simulink model "FinalmodelMad2Order"  (R2022b)
settings: Solver=FixedStepAuto  StartTime=0.0  StopTime=inf  RelTol=1e-3  EnableMultiTasking=on
libraries: vexarmcortexlib x25, vexcommonlib x1
settings Model: ExtModeTrigDuration=25  Creator=Mihai Nicoara  LastModifiedBy=bobsi
settings SolverCC: AutoInsertRateTranBlk=on
settings OptimizationCC: EnhancedBackFolding=on  PassReuseOutputArgsAs=Individual arguments  ZeroExternalMemoryAtStartup=off  ZeroInternalMemoryAtStartup=off  MaxStackSize=64  OptimizeBlockOrder=speed  DifferentSizesBufferReuse=on  OptimizationCustomize=off  EfficientTunableParamExpr=on
settings DebuggingCC: ParameterTunabilityLossMsg=error
settings HardwareCC: ProdBitPerPointer=32  ProdBitPerSizeT=32  ProdBitPerPtrDiffT=32  ProdLargestAtomicInteger=Long  ProdLargestAtomicFloat=Double  ProdWordSize=32  ProdHWDeviceType=ARM Compatible->ARM Cortex
settings SFSimCC: MATLABDynamicMemAlloc=off
settings RTWCC: Description=Embedded Coder  SystemTargetFile=ert.tlc  HardwareBoard=ARM Cortex-based VEX Microcontroller  TLCOptions="-aInlineSetEventsForThisBaseRateFcn=TLC_FALSE -aSuppressMultiTaskScheduler=TLC_FALSE  -aRateBasedStepFcn=0"  TemplateMakefile=ert_default_tmf  Toolchain=GNU Tools for VEX ARM Cortex
settings CodeAppCC: ForceParamTrailComments=on  IgnoreCustomStorageClasses=off  OperatorAnnotations=on  SimulinkDataObjDesc=on  SFDataObjDesc=on  InsertBlockDesc=on
settings ERTTargetCC: ExtModeTransport=1  ExtModeMexFile=ext_serial_win32_comm

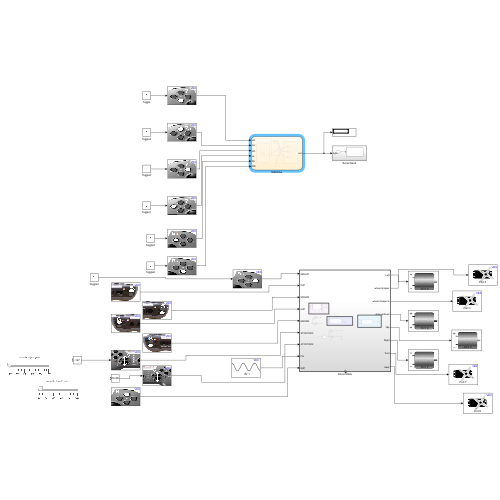
[thumbnail: Simulink's stored preview of the top-level diagram]
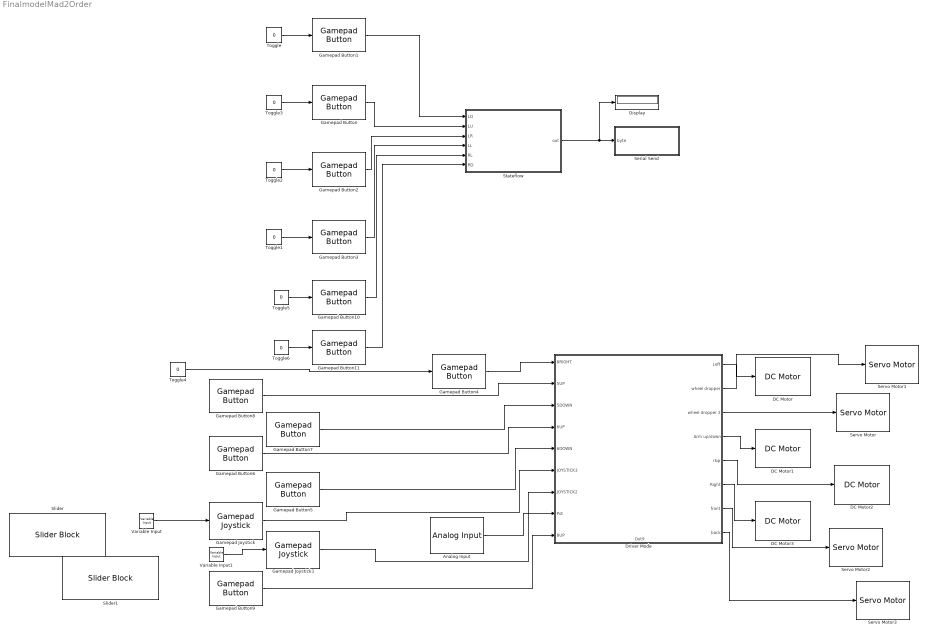
== system FinalmodelMad2Order ==
  Analog Input : vexarmcortexlib/Sensors/Analog Input  inChan=1  SimulationIn=off  SampleTime=0.02
  DC Motor : vexarmcortexlib/Actuators/DC Motor  motor=9  scaleFactor=1/13.5  SimulationOut=off
  DC Motor1 : vexarmcortexlib/Actuators/DC Motor  motor=4  scaleFactor=1/13.5  SimulationOut=off
  DC Motor2 : vexarmcortexlib/Actuators/DC Motor  motor=6  scaleFactor=1/13.5  SimulationOut=off
  DC Motor3 : vexarmcortexlib/Actuators/DC Motor  motor=2  scaleFactor=1/13.5  SimulationOut=off
  Display : Display
  Driver Mode : Subsystem  TreatAsAtomicUnit=on
      settings: PortSchema="{\"entries\":[{\"content\":{\"sides\":[{\"content\":{\"connectorIds\":[\"In1\",\"In2\",\"In3\",\"In4\",\"In5\",\"In6\",\"In7\",\"In8\",\"In9\"]},\"type\":\"ConnectorPlacement.EquallySpacedRectSide\",\"uuid\":\"20c58c0e-6097-4e33-992f-9b990da3c46e\"},{\"content\":{\"connectorIds\":[\"Out1\",\"Out2\",\"Out3\",\"Out4\",\"Out5\",\"Out6\",\"Out7\",\"Out8\"],\"side\":\"RIGHT\"},\"type\":\"ConnectorPlacement.EquallySpacedRectSide\",\"uuid\":\"672ab42f-08c0-4fe5-8585-267d7f24fa0b\"},{\"content\":{\"connectorIds\":[],\"side\":\"TOP\"},\"type\":\"ConnectorPlacement.EquallySpacedRectSide\",\"uuid\":\"0be9b8b5-8d19-40cb-8006-b33ff3da0e45\"},{\"content\":{\"connectorIds\":[\"Out9\"],\"side\":\"BOTTOM\"},\"type\":\"ConnectorPlacement.EquallySpacedRectSide\",\"uuid\":\"bbd838f8-255e-4ffd-82e4-fbeb741872fd\"}]},\"type\":\"ConnectorPlacement.EquallySpacedConnector\",\"uuid\":\"2462ad6d-f70b-4cc9-a378-cd07eeaa0f93\"}],\"packageUris\":[\"http://schema.mathworks.com/mf0/Connector/R2020b\"],\"version\":\"1.0\"}"
  Gamepad Button : vexarmcortexlib/Gamepad/Gamepad Button  joystick=1  chan=7  button56=Up  button78=Up  SimulationIn=on  SampleTime=0.02
  Gamepad Button1 : vexarmcortexlib/Gamepad/Gamepad Button  joystick=1  chan=7  button56=Up  button78=Down  SimulationIn=on  SampleTime=0.02
  Gamepad Button10 : vexarmcortexlib/Gamepad/Gamepad Button  joystick=1  chan=8  button56=Up  button78=Left  SimulationIn=on  SampleTime=0.02
  Gamepad Button11 : vexarmcortexlib/Gamepad/Gamepad Button  joystick=1  chan=8  button56=Up  button78=Down  SimulationIn=on  SampleTime=0.02
  Gamepad Button2 : vexarmcortexlib/Gamepad/Gamepad Button  joystick=1  chan=7  button56=Up  button78=Right  SimulationIn=on  SampleTime=0.02
  Gamepad Button3 : vexarmcortexlib/Gamepad/Gamepad Button  joystick=1  chan=7  button56=Up  button78=Left  SimulationIn=on  SampleTime=0.02
  Gamepad Button4 : vexarmcortexlib/Gamepad/Gamepad Button  joystick=1  chan=8  button56=Up  button78=Right  SimulationIn=on  SampleTime=0.02
  Gamepad Button5 : vexarmcortexlib/Gamepad/Gamepad Button  joystick=1  chan=6  button56=Down  button78=Left  SimulationIn=off  SampleTime=0.02
  Gamepad Button6 : vexarmcortexlib/Gamepad/Gamepad Button  joystick=1  chan=6  button56=Up  button78=Left  SimulationIn=off  SampleTime=0.02
  Gamepad Button7 : vexarmcortexlib/Gamepad/Gamepad Button  joystick=1  chan=5  button56=Down  button78=Left  SimulationIn=off  SampleTime=0.02
  Gamepad Button8 : vexarmcortexlib/Gamepad/Gamepad Button  joystick=1  chan=5  button56=Up  button78=Left  SimulationIn=off  SampleTime=0.02
  Gamepad Button9 : vexarmcortexlib/Gamepad/Gamepad Button  joystick=1  chan=8  button56=Down  button78=Up  SimulationIn=off  SampleTime=0.02
  Gamepad Joystick : vexarmcortexlib/Gamepad/Gamepad Joystick  joystick=1  chan=3  SimulationIn=on  SampleTime=0.02
  Gamepad Joystick1 : vexarmcortexlib/Gamepad/Gamepad Joystick  joystick=1  chan=2  SimulationIn=on  SampleTime=0.02
  Serial Send : Subsystem
  Servo Motor : vexarmcortexlib/Actuators/Servo Motor  motor=3  scaleFactor=60/127  SimulationOut=off
  Servo Motor1 : vexarmcortexlib/Actuators/Servo Motor  motor=5  scaleFactor=60/127  SimulationOut=off
  Servo Motor2 : vexarmcortexlib/Actuators/Servo Motor  motor=7  scaleFactor=60/127  SimulationOut=off
  Servo Motor3 : vexarmcortexlib/Actuators/Servo Motor  motor=8  scaleFactor=60/127  SimulationOut=off
  Slider : SliderBlock  ScaleMin=-127  ScaleMax=127
  Slider1 : SliderBlock  ScaleMin=-127  ScaleMax=127
  Stateflow : Stateflow chart  TreatAsAtomicUnit=on
  Toggle{,1..6} (7 alike) : Constant  Value=0
      settings: OpenFcn=|
      | if strcmp('0',get_param(gcb, 'Value'))                        set_param(gcb, 'Value', '1');
      | else
      |             set_param(gcb, 'Value', '0');
      | end
  Variable Input : vexarmcortexlib/Utilities/Variable Input  low=-127  gain=-127  high=127
  Variable Input1 : vexarmcortexlib/Utilities/Variable Input  low=-127  gain=-109.4937343358396  high=127
  wires:
  Gamepad Button/1 -> Stateflow/2(LU)
  Stateflow/1(out) -> Display/1, Serial Send/1(byte)
  Gamepad Button2/1 -> Stateflow/3(LR)
  Gamepad Button3/1 -> Stateflow/4(LL)
  Gamepad Button1/1 -> Stateflow/1(LD)
  Toggle/1 -> Gamepad Button1/1
  Toggle3/1 -> Gamepad Button/1
  Toggle2/1 -> Gamepad Button2/1
  Toggle1/1 -> Gamepad Button3/1
  Gamepad Button4/1 -> Driver Mode/1(8RIGHT)
  Gamepad Button8/1 -> Driver Mode/2(5UP)
  Gamepad Button7/1 -> Driver Mode/3(5DOWN)
  Gamepad Button6/1 -> Driver Mode/4(6UP)
  Gamepad Button5/1 -> Driver Mode/5(6DOWN)
  Gamepad Joystick/1 -> Driver Mode/6(JOYSTICK3)
  Gamepad Joystick1/1 -> Driver Mode/7(JOYSTICK2)
  Driver Mode/1(Left) -> DC Motor/1
  Driver Mode/6(Right) -> DC Motor3/1
  Driver Mode/4(Arm up/down) -> DC Motor1/1
  Driver Mode/3(wheel dropper 2) -> Servo Motor/1
  Driver Mode/5(r&p) -> DC Motor2/1
  Analog Input/1 -> Driver Mode/8(Pot)
  Toggle4/1 -> Gamepad Button4/1
  Driver Mode/2(wheel dropper) -> Servo Motor1/1
  Driver Mode/7(front) -> Servo Motor2/1
  Driver Mode/8(back) -> Servo Motor3/1
  Gamepad Button9/1 -> Driver Mode/9(8UP)
  Toggle5/1 -> Gamepad Button10/1
  Variable Input1/1 -> Gamepad Joystick1/1
  Variable Input/1 -> Gamepad Joystick/1
  Gamepad Button10/1 -> Stateflow/5(RL)
  Toggle6/1 -> Gamepad Button11/1
  Gamepad Button11/1 -> Stateflow/6(RD)

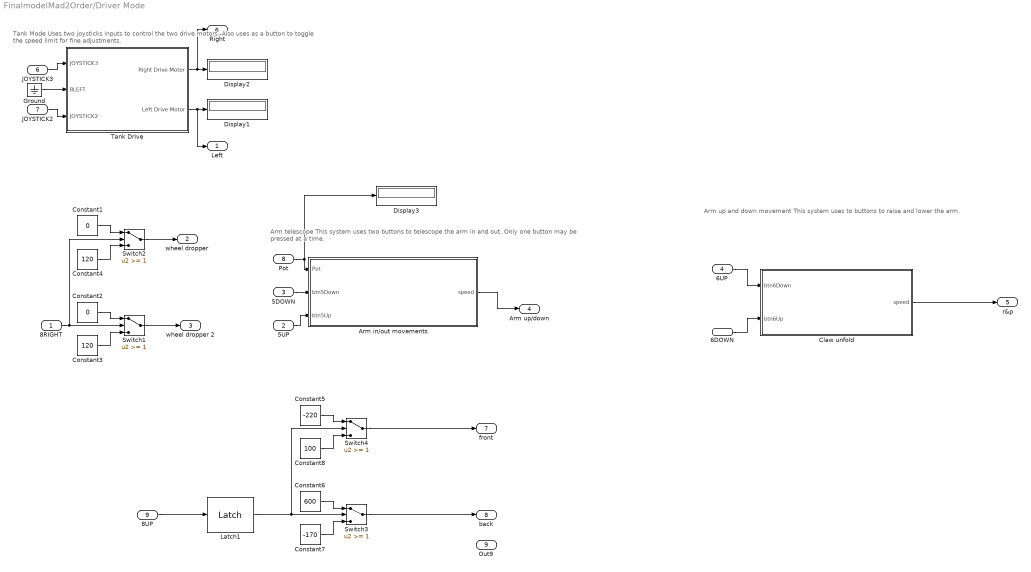
== system FinalmodelMad2Order/Driver Mode ==
  note: Tank Mode
      | Uses two joysticks inputs to control the two drive motors. Also uses as a button
      | to toggle the speed limit for fine adjustments.
  note: Arm up and down movement
      | This system uses to buttons to raise and lower the arm.
  note: Arm telescope
      | This system uses two buttons to telescope the arm in and out.
      | Only one button may be pressed at a time.
  8RIGHT : Inport
  5UP : Inport  Port=2
  5DOWN : Inport  Port=3
  6UP : Inport  Port=4
  6DOWN : Inport  Port=5
  JOYSTICK3 : Inport  Port=6
  JOYSTICK2 : Inport  Port=7
  Pot : Inport  Port=8
  8UP : Inport  Port=9
  Arm in/out movements : Stateflow chart  TreatAsAtomicUnit=on
  Claw unfold : Stateflow chart  TreatAsAtomicUnit=on
  Constant1 : Constant  Value=0
  Constant2 : Constant  Value=0
  Constant3 : Constant  Value=120
  Constant4 : Constant  Value=120
  Constant5 : Constant  Value=-220
  Constant6 : Constant  Value=600
  Constant7 : Constant  Value=-170
  Constant8 : Constant  Value=100
  Display1 : Display
  Display2 : Display
  Display3 : Display
  Ground : Ground
  Latch1 : vexcommonlib/Latch  output0=off  BlockPlatform=vexarmcortex
      settings: LibrarySourceBlock=vexarmcortexlib/Utilities/Latch
  Switch{1..4} (4 alike) : Switch  Threshold=1  SaturateOnIntegerOverflow=off  InputSameDT=off
  "Tank Drive " : Subsystem  TreatAsAtomicUnit=on
  Left : Outport
  wheel dropper : Outport  Port=2
  wheel dropper 2 : Outport  Port=3
  Arm up/down : Outport  Port=4
  r&p : Outport  Port=5
  Right : Outport  Port=6
  front : Outport  Port=7
  back : Outport  Port=8
  Out9 : Outport  Port=9
  wires:
  Claw unfold/1(speed) -> r&p/1
  "Tank Drive "/2(Left Drive Motor) -> Left/1, Display1/1
  "Tank Drive "/1(Right Drive Motor) -> Right/1, Display2/1
  JOYSTICK2/1 -> "Tank Drive "/3(JOYSTICK2)
  JOYSTICK3/1 -> "Tank Drive "/1(JOYSTICK3)
  Arm in/out movements/1(speed) -> Arm up/down/1
  6UP/1 -> Claw unfold/1(btn6Down)
  6DOWN/1 -> Claw unfold/2(btn6Up)
  5UP/1 -> Arm in/out movements/3(btn5Up)
  5DOWN/1 -> Arm in/out movements/2(btn5Down)
  Pot/1 -> Arm in/out movements/1(Pot), Display3/1
  Constant2/1 -> Switch1/1
  Constant3/1 -> Switch1/3
  Switch1/1 -> wheel dropper 2/1
  Constant4/1 -> Switch2/3
  8RIGHT/1 -> Switch2/2, Switch1/2
  Switch2/1 -> wheel dropper/1
  Constant1/1 -> Switch2/1
  Constant5/1 -> Switch4/1
  Constant8/1 -> Switch4/3
  Constant6/1 -> Switch3/1
  8UP/1 -> Latch1/1
  Constant7/1 -> Switch3/3
  Switch4/1 -> front/1
  Switch3/1 -> back/1
  Latch1/1 -> Switch4/2, Switch3/2
  Ground/1 -> "Tank Drive "/2(8LEFT)

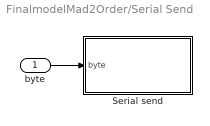
== system FinalmodelMad2Order/Serial Send ==
  byte : Inport  OutDataTypeStr=uint8  PortDimensions=[1 1]
  Serial send : MATLAB Function  TreatAsAtomicUnit=on
  wires:
  byte/1 -> Serial send/1(byte)

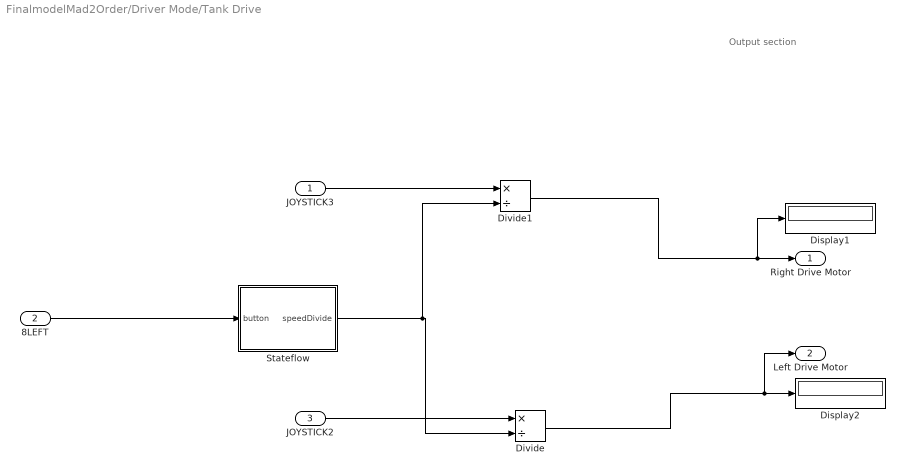
== system FinalmodelMad2Order/Driver Mode/Tank Drive  ==
  note: Output section
  JOYSTICK3 : Inport
  8LEFT : Inport  Port=2
  JOYSTICK2 : Inport  Port=3
  Display1 : Display
  Display2 : Display
  Divide : Product  Inputs=*/
  Divide1 : Product  Inputs=*/
  Stateflow : Stateflow chart  TreatAsAtomicUnit=on
  Right Drive Motor : Outport
  Left Drive Motor : Outport  Port=2
  wires:
  Divide/1 -> Left Drive Motor/1, Display2/1
  8LEFT/1 -> Stateflow/1(button)
  Divide1/1 -> Display1/1, Right Drive Motor/1
  JOYSTICK2/1 -> Divide/1
  Stateflow/1(speedDivide) -> Divide1/2, Divide/2
  JOYSTICK3/1 -> Divide1/1

== stateflow chart FinalmodelMad2Order/Driver Mode/Arm in//out movements ==
  state ARMDOWN
    entry:
    speed = -70;
  state STOPPED
    entry:
    speed = 20;
  state ARMUP
    entry:
    speed = 80;
  (default) -> STOPPED
  STOPPED -> ARMUP [order 1] : [btn5Down == 0 && btn5Up == 1 ]
  STOPPED -> ARMDOWN [order 2] : [btn5Down == 1 && btn5Up == 0]
  ARMDOWN -> STOPPED : [btn5Down == 0]
  ARMUP -> STOPPED : [btn5Up == 0]
  data: Pot input; btn5Down input; btn5Up input; speed output

== stateflow chart FinalmodelMad2Order/Driver Mode/Claw unfold ==
  state ARMDOWN
    entry:
    speed = -140;
  state STOPPED
    entry:
    speed = 0;
  state ARMUP
    entry:
    speed = 140;
  (default) -> STOPPED
  STOPPED -> ARMUP [order 1] : [btn6Down == 0 && btn6Up == 1 ]
  STOPPED -> ARMDOWN [order 2] : [btn6Down == 1 && btn6Up == 0]
  ARMDOWN -> STOPPED [order 2] : [btn6Down == 0]
  ARMUP -> STOPPED [order 2] : [btn6Up == 0]
  ARMDOWN -> STOPPED [order 1] : [btn6Down == 1 && btn6Up == 1]
  ARMUP -> STOPPED [order 1] : [btn6Down == 1 && btn6Up == 1]
  data: speed output; btn6Down input; btn6Up input

== stateflow chart FinalmodelMad2Order/Stateflow ==
  state Speed Adjustments [group]
    state speedHigh
      entry:
      out = 0xC3;
  state Squeaky Movements [group]
    state LiftMid
      entry:
      out = 0x66;
    state driveRight
      entry:
      out = 0x5A;
    state rotateRight
      entry:
      out = 0x3C;
  state Rotational Adjustments [group]
    state RotHigh
      entry:
      out = 0x0F;
  state Default_Flash
    entry:
    out = 0xF0;
  state MasterFeildReset
    entry:
    out = 0xAA;
  Default_Flash -> speedHigh [order 4] : [RL == 1]
  speedHigh -> Default_Flash : [after(0.5,sec)]
  Default_Flash -> LiftMid [order 1] : [LL == 1]
  LiftMid -> Default_Flash : [after(0.5,sec)]
  (default) -> Default_Flash
  Default_Flash -> RotHigh [order 5] : [RD == 1]
  RotHigh -> Default_Flash : [after(0.5,sec)]
  Default_Flash -> MasterFeildReset [order 6] : [LU == 1 && LD == 1 && LR == 1 && LL == 1]
  MasterFeildReset -> Default_Flash : [after(0.5,sec)]
  rotateRight -> Default_Flash : [after(0.5,sec)]
  Default_Flash -> rotateRight [order 3] : [LR == 1]
  driveRight -> Default_Flash : [after(0.5,sec)]
  Default_Flash -> driveRight [order 2] : [LD == 1]
  data: LD input; LU input; out output; LR input; LL input; RL input; RD input

== stateflow chart FinalmodelMad2Order/Driver Mode/Tank Drive /Stateflow ==
  state Slow_Speed
    entry:
    speedDivide = 2;
  state Full_Speed
    entry:
    speedDivide = 1;
  (default) -> Full_Speed
  Full_Speed -> Slow_Speed : [button == 1]
  Slow_Speed -> Full_Speed : [button == 0]
  data: speedDivide output; button input

== matlab function FinalmodelMad2Order/Serial Send/Serial send ==
  data: byte input
function fcn(byte)
% Serial send single byte
%#codegen

% Config
port = 'uart1';
baud = uint32(600);

persistent isFirstRun

if coder.target('Rtw')
    coder.cinclude('API.h');
    coder.cinclude('string.h');
    file = coder.opaque('FILE *', port,'HeaderFile','API.h');

    if isempty(isFirstRun)
        % first time setup
        isFirstRun = false;

        flags = coder.opaque('uint16', 'SERIAL_8N1');
        coder.ceval('usartInit', file, baud, flags);
    end

    coder.ceval('fputc', byte, file);

end

end
